simulink model "EKF"  (R2023b)
settings: Solver=FixedStepAuto  StartTime=tstart  StopTime=tend  FixedStep=0.1  RelTol=1e-3
values from neighbouring files (symbols this model uses):
  EKF_P0 = eye(7)    [main_script.m]
  inertia_p = [85.075, 0, 0; 0, 85.075, 0; 0, 0, 120.2515]    [omega_dot.m]
settings Model: Creator=Anna  LastModifiedBy=Ethan

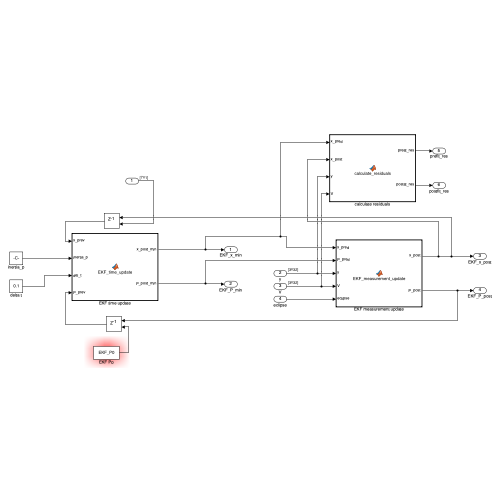
[thumbnail: Simulink's stored preview of the top-level diagram]
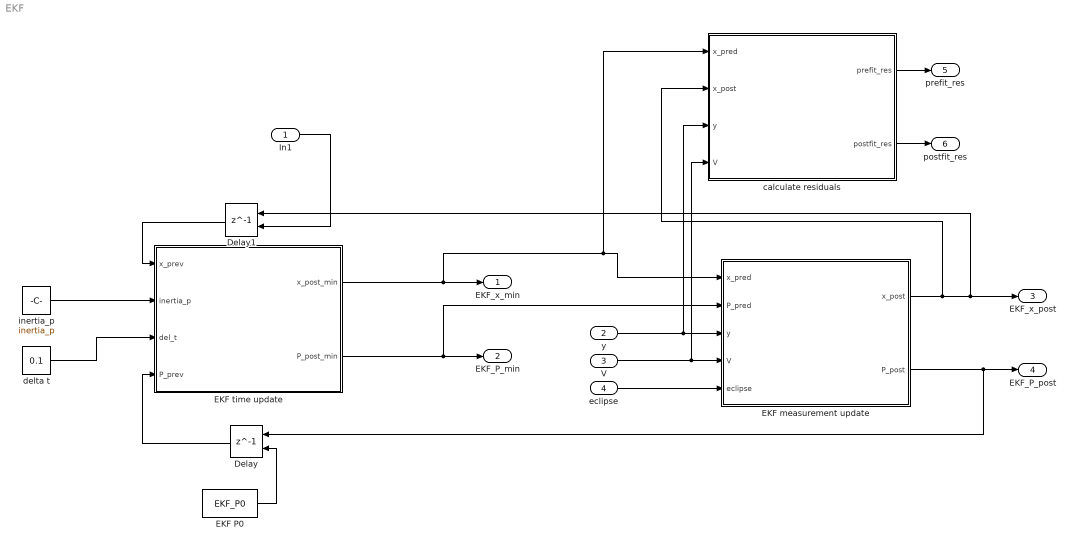
== system EKF ==
  In1 : Inport  PortDimensions=[7 1]
  y : Inport  Port=2  PortDimensions=[3, 32]
  V : Inport  Port=3  PortDimensions=[3, 32]
  eclipse : Inport  Port=4
  Delay : Delay  DelayLength=1  InitialConditionSource=Input port  InitialCondition=0
      settings: InputPortMap=u0,p4
  Delay1 : Delay  DelayLength=1  InitialConditionSource=Input port  InitialCondition=0
      settings: InputPortMap=u0,p4
  EKF P0 : Constant  Value=EKF_P0
  EKF measurement update : MATLAB Function  TreatAsAtomicUnit=on
  EKF time update : MATLAB Function  TreatAsAtomicUnit=on
  calculate residuals : MATLAB Function  TreatAsAtomicUnit=on
  delta t : Constant  Value=0.1
  inertia_p : Constant  Value=inertia_p
  EKF_x_min : Outport
  EKF_P_min : Outport  Port=2
  EKF_x_post : Outport  Port=3
  EKF_P_post : Outport  Port=4
  prefit_res : Outport  Port=5
  postfit_res : Outport  Port=6
  wires:
  Delay1/1 -> EKF time update/1(x_prev)
  In1/1 -> Delay1/2
  Delay/1 -> EKF time update/4(P_prev)
  EKF time update/1(x_post_min) -> calculate residuals/1(x_pred), EKF measurement update/1(x_pred), EKF_x_min/1
  EKF time update/2(P_post_min) -> EKF measurement update/2(P_pred), EKF_P_min/1
  EKF P0/1 -> Delay/2
  inertia_p/1 -> EKF time update/2(inertia_p)
  delta t/1 -> EKF time update/3(del_t)
  EKF measurement update/1(x_post) -> calculate residuals/2(x_post), Delay1/1, EKF_x_post/1
  EKF measurement update/2(P_post) -> Delay/1, EKF_P_post/1
  y/1 -> calculate residuals/3(y), EKF measurement update/3(y)
  V/1 -> calculate residuals/4(V), EKF measurement update/4(V)
  eclipse/1 -> EKF measurement update/5(eclipse)
  calculate residuals/1(prefit_res) -> prefit_res/1
  calculate residuals/2(postfit_res) -> postfit_res/1

== matlab function EKF/EKF measurement update ==
  data: x_pred input; P_pred input; y input; x_post output; P_post output; V input; eclipse input
function [x_post, P_post] = EKF_measurement_update(x_pred, P_pred, y, V, eclipse)

    

    %Sun
    if 1 %~eclipse
        rx = V(1, 1);
        ry = V(2, 1);
        rz = V(3, 1);
        q1 = x_pred(4);
        q2 = x_pred(5);
        q3 = x_pred(6);
        q4 = x_pred(7);
        
        %DCM 
        DCM = [q1^2 - q2^2 - q3^2 + q4^2, 2*q1*q2 + 2*q3*q4, 2*q1*q3 - 2*q2*q4;
            2*q1*q2 - 2*q3*q4, -q1^2 + q2^2 - q3^2 + q4^2, 2*q1*q4 + 2*q2*q3;
            2*q1*q3 + 2*q2*q4, 2*q2*q3 - 2*q1*q4, -q1^2 - q2^2 + q3^2 + q4^2];

        %Sensitivity Matrix
        H = [0, 0, 0, 2*q1*rx + 2*q2*ry + 2*q3*rz, -2*q2*rx + 2*q1*ry - 2*q4*rz, -2*q3*rx + 2*q4*ry + 2*q1*rz,  2*q4*rx + 2*q3*ry - 2*q2*rz;
            0, 0, 0, 2*q2*rx - 2*q1*ry + 2*q4*rz,  2*q1*rx + 2*q2*ry + 2*q3*rz, -2*q4*rx - 2*q3*ry + 2*q2*rz, -2*q3*rx + 2*q4*ry + 2*q1*rz;
            0, 0, 0, 2*q3*rx - 2*q4*ry - 2*q1*rz,  2*q4*rx + 2*q3*ry - 2*q2*rz,  2*q1*rx + 2*q2*ry + 2*q3*rz,  2*q2*rx - 2*q1*ry + 2*q4*rz];
        %Kalman Gain
        R = 0.13913 * eye(3);
        S = H * P_pred * H' + R;
        K = (P_pred * H')/(S); %nxm

        %disp(y(:, 1) - H * x_pred)
        x_pred = x_pred + K * (y(:, 1) -  DCM * V(:, 1));
        P_pred = (eye(length(x_pred), length(x_pred)) - K * H) * P_pred *(eye(length(x_pred), length(x_pred)))' + K*R*K';
 
    end
    
    %Magnetic
    rx = V(1, 2);
    ry = V(2, 2);
    rz = V(3, 2);
    q1 = x_pred(4);
    q2 = x_pred(5);
    q3 = x_pred(6);
    q4 = x_pred(7);

    %DCM 
    DCM = [q1^2 - q2^2 - q3^2 + q4^2, 2*q1*q2 + 2*q3*q4, 2*q1*q3 - 2*q2*q4;
            2*q1*q2 - 2*q3*q4, -q1^2 + q2^2 - q3^2 + q4^2, 2*q1*q4 + 2*q2*q3;
            2*q1*q3 + 2*q2*q4, 2*q2*q3 - 2*q1*q4, -q1^2 - q2^2 + q3^2 + q4^2];

    %Sensitivity Matrix
    H = [0, 0, 0, 2*q1*rx + 2*q2*ry + 2*q3*rz, -2*q2*rx + 2*q1*ry - 2*q4*rz, -2*q3*rx + 2*q4*ry + 2*q1*rz,  2*q4*rx + 2*q3*ry - 2*q2*rz;
        0, 0, 0, 2*q2*rx - 2*q1*ry + 2*q4*rz,  2*q1*rx + 2*q2*ry + 2*q3*rz, -2*q4*rx - 2*q3*ry + 2*q2*rz, -2*q3*rx + 2*q4*ry + 2*q1*rz;
        0, 0, 0, 2*q3*rx - 2*q4*ry - 2*q1*rz,  2*q4*rx + 2*q3*ry - 2*q2*rz,  2*q1*rx + 2*q2*ry + 2*q3*rz,  2*q2*rx - 2*q1*ry + 2*q4*rz];
    %Kalman Gain
    R =  3.05974 * 1e-7 * eye(3);
    S = H * P_pred * H' + R;
    K = (P_pred * H') / S; %nxm

    x_pred = x_pred + K * (y(:, 2) - DCM * V(:, 2));
    P_pred = (eye(length(x_pred), length(x_pred)) - K * H) * P_pred *(eye(length(x_pred), length(x_pred)))' + K*R*K';

    %Star
    for i = 3:32
        rx = V(1, i);
        ry = V(2, i);
        rz = V(3, i);
        q1 = x_pred(4);
        q2 = x_pred(5);
        q3 = x_pred(6);
        q4 = x_pred(7);


        %DCM 
        DCM = [q1^2 - q2^2 - q3^2 + q4^2, 2*q1*q2 + 2*q3*q4, 2*q1*q3 - 2*q2*q4;
                2*q1*q2 - 2*q3*q4, -q1^2 + q2^2 - q3^2 + q4^2, 2*q1*q4 + 2*q2*q3;
                2*q1*q3 + 2*q2*q4, 2*q2*q3 - 2*q1*q4, -q1^2 - q2^2 + q3^2 + q4^2];

        %Sensitivity Matrix
        H = [0, 0, 0, 2*q1*rx + 2*q2*ry + 2*q3*rz, -2*q2*rx + 2*q1*ry - 2*q4*rz, -2*q3*rx + 2*q4*ry + 2*q1*rz,  2*q4*rx + 2*q3*ry - 2*q2*rz;
            0, 0, 0, 2*q2*rx - 2*q1*ry + 2*q4*rz,  2*q1*rx + 2*q2*ry + 2*q3*rz, -2*q4*rx - 2*q3*ry + 2*q2*rz, -2*q3*rx + 2*q4*ry + 2*q1*rz;
            0, 0, 0, 2*q3*rx - 2*q4*ry - 2*q1*rz,  2*q4*rx + 2*q3*ry - 2*q2*rz,  2*q1*rx + 2*q2*ry + 2*q3*rz,  2*q2*rx - 2*q1*ry + 2*q4*rz];
        %Kalman Gain
        R = 2.342 * 1e-7 * eye(3);
        S = H * P_pred * H' + R;
        K = (P_pred * H') / S; %nxm



        x_pred = x_pred + K * (y(:, i) -  DCM * V(:, i));
        P_pred = (eye(length(x_pred), length(x_pred)) - K * H) * P_pred *(eye(length(x_pred), length(x_pred)))' + K*R*K';
    end
    
    x_post = x_pred;
    x_post(4:end) = x_post(4:end)./norm(x_post(4:end));
    P_post = P_pred;

== matlab function EKF/calculate residuals ==
  data: x_pred input; x_post input; prefit_res output; postfit_res output; y input; V input
function [prefit_res, postfit_res] = calculate_residuals(x_pred, x_post, y, V)
    prefit_res = zeros(3, 3);
    postfit_res = zeros(3, 3);
    
    %% Prefit
    q1 = x_pred(4);
    q2 = x_pred(5);
    q3 = x_pred(6);
    q4 = x_pred(7);

    rx = V(1, 1);
    ry = V(2, 1);
    rz = V(3, 1);

    %% Sun
    %DCM 
    DCM = [q1^2 - q2^2 - q3^2 + q4^2, 2*q1*q2 + 2*q3*q4, 2*q1*q3 - 2*q2*q4;
        2*q1*q2 - 2*q3*q4, -q1^2 + q2^2 - q3^2 + q4^2, 2*q1*q4 + 2*q2*q3;
        2*q1*q3 + 2*q2*q4, 2*q2*q3 - 2*q1*q4, -q1^2 - q2^2 + q3^2 + q4^2];

    %Sensitivity Matrix
    H = [0, 0, 0, 2*q1*rx + 2*q2*ry + 2*q3*rz, -2*q2*rx + 2*q1*ry - 2*q4*rz, -2*q3*rx + 2*q4*ry + 2*q1*rz,  2*q4*rx + 2*q3*ry - 2*q2*rz;
        0, 0, 0, 2*q2*rx - 2*q1*ry + 2*q4*rz,  2*q1*rx + 2*q2*ry + 2*q3*rz, -2*q4*rx - 2*q3*ry + 2*q2*rz, -2*q3*rx + 2*q4*ry + 2*q1*rz;
        0, 0, 0, 2*q3*rx - 2*q4*ry - 2*q1*rz,  2*q4*rx + 2*q3*ry - 2*q2*rz,  2*q1*rx + 2*q2*ry + 2*q3*rz,  2*q2*rx - 2*q1*ry + 2*q4*rz];
    %Kalman Gain
    prefit_res(:, 1) = y(:, 1) -  DCM * V(:, 1);

    
    %Magnetic
    rx = V(1, 2);
    ry = V(2, 2);
    rz = V(3, 2);

    %DCM 
    DCM = [q1^2 - q2^2 - q3^2 + q4^2, 2*q1*q2 + 2*q3*q4, 2*q1*q3 - 2*q2*q4;
            2*q1*q2 - 2*q3*q4, -q1^2 + q2^2 - q3^2 + q4^2, 2*q1*q4 + 2*q2*q3;
            2*q1*q3 + 2*q2*q4, 2*q2*q3 - 2*q1*q4, -q1^2 - q2^2 + q3^2 + q4^2];

    %Sensitivity Matrix
    H = [0, 0, 0, 2*q1*rx + 2*q2*ry + 2*q3*rz, -2*q2*rx + 2*q1*ry - 2*q4*rz, -2*q3*rx + 2*q4*ry + 2*q1*rz,  2*q4*rx + 2*q3*ry - 2*q2*rz;
        0, 0, 0, 2*q2*rx - 2*q1*ry + 2*q4*rz,  2*q1*rx + 2*q2*ry + 2*q3*rz, -2*q4*rx - 2*q3*ry + 2*q2*rz, -2*q3*rx + 2*q4*ry + 2*q1*rz;
        0, 0, 0, 2*q3*rx - 2*q4*ry - 2*q1*rz,  2*q4*rx + 2*q3*ry - 2*q2*rz,  2*q1*rx + 2*q2*ry + 2*q3*rz,  2*q2*rx - 2*q1*ry + 2*q4*rz];
    %Kalman Gain
    prefit_res(:, 2) = y(:, 2) -  DCM * V(:, 2);

    %Star
    star_residuals = zeros(3, 30);
    for i = 3:32
        rx = V(1, i);
        ry = V(2, i);
        rz = V(3, i);


        %DCM 
        DCM = [q1^2 - q2^2 - q3^2 + q4^2, 2*q1*q2 + 2*q3*q4, 2*q1*q3 - 2*q2*q4;
                2*q1*q2 - 2*q3*q4, -q1^2 + q2^2 - q3^2 + q4^2, 2*q1*q4 + 2*q2*q3;
                2*q1*q3 + 2*q2*q4, 2*q2*q3 - 2*q1*q4, -q1^2 - q2^2 + q3^2 + q4^2];

        %Sensitivity Matrix
        H = [0, 0, 0, 2*q1*rx + 2*q2*ry + 2*q3*rz, -2*q2*rx + 2*q1*ry - 2*q4*rz, -2*q3*rx + 2*q4*ry + 2*q1*rz,  2*q4*rx + 2*q3*ry - 2*q2*rz;
            0, 0, 0, 2*q2*rx - 2*q1*ry + 2*q4*rz,  2*q1*rx + 2*q2*ry + 2*q3*rz, -2*q4*rx - 2*q3*ry + 2*q2*rz, -2*q3*rx + 2*q4*ry + 2*q1*rz;
            0, 0, 0, 2*q3*rx - 2*q4*ry - 2*q1*rz,  2*q4*rx + 2*q3*ry - 2*q2*rz,  2*q1*rx + 2*q2*ry + 2*q3*rz,  2*q2*rx - 2*q1*ry + 2*q4*rz];
        %Kalman Gain
        star_residuals(:, i-2) = y(:, i) -  DCM * V(:, i);

    end
    prefit_res(:, 3) = mean(star_residuals, 2);

    %% Post fit

    q1 = x_post(4);
    q2 = x_post(5);
    q3 = x_post(6);
    q4 = x_post(7);
    %% Sun
    %DCM 
    DCM = [q1^2 - q2^2 - q3^2 + q4^2, 2*q1*q2 + 2*q3*q4, 2*q1*q3 - 2*q2*q4;
        2*q1*q2 - 2*q3*q4, -q1^2 + q2^2 - q3^2 + q4^2, 2*q1*q4 + 2*q2*q3;
        2*q1*q3 + 2*q2*q4, 2*q2*q3 - 2*q1*q4, -q1^2 - q2^2 + q3^2 + q4^2];

    %Sensitivity Matrix
    H = [0, 0, 0, 2*q1*rx + 2*q2*ry + 2*q3*rz, -2*q2*rx + 2*q1*ry - 2*q4*rz, -2*q3*rx + 2*q4*ry + 2*q1*rz,  2*q4*rx + 2*q3*ry - 2*q2*rz;
        0, 0, 0, 2*q2*rx - 2*q1*ry + 2*q4*rz,  2*q1*rx + 2*q2*ry + 2*q3*rz, -2*q4*rx - 2*q3*ry + 2*q2*rz, -2*q3*rx + 2*q4*ry + 2*q1*rz;
        0, 0, 0, 2*q3*rx - 2*q4*ry - 2*q1*rz,  2*q4*rx + 2*q3*ry - 2*q2*rz,  2*q1*rx + 2*q2*ry + 2*q3*rz,  2*q2*rx - 2*q1*ry + 2*q4*rz];
    %Kalman Gain
    postfit_res(:, 1) = y(:, 1) -  DCM * V(:, 1);

    
    %Magnetic
    rx = V(1, 2);
    ry = V(2, 2);
    rz = V(3, 2);

    %DCM 
    DCM = [q1^2 - q2^2 - q3^2 + q4^2, 2*q1*q2 + 2*q3*q4, 2*q1*q3 - 2*q2*q4;
            2*q1*q2 - 2*q3*q4, -q1^2 + q2^2 - q3^2 + q4^2, 2*q1*q4 + 2*q2*q3;
            2*q1*q3 + 2*q2*q4, 2*q2*q3 - 2*q1*q4, -q1^2 - q2^2 + q3^2 + q4^2];

    %Sensitivity Matrix
    H = [0, 0, 0, 2*q1*rx + 2*q2*ry + 2*q3*rz, -2*q2*rx + 2*q1*ry - 2*q4*rz, -2*q3*rx + 2*q4*ry + 2*q1*rz,  2*q4*rx + 2*q3*ry - 2*q2*rz;
        0, 0, 0, 2*q2*rx - 2*q1*ry + 2*q4*rz,  2*q1*rx + 2*q2*ry + 2*q3*rz, -2*q4*rx - 2*q3*ry + 2*q2*rz, -2*q3*rx + 2*q4*ry + 2*q1*rz;
        0, 0, 0, 2*q3*rx - 2*q4*ry - 2*q1*rz,  2*q4*rx + 2*q3*ry - 2*q2*rz,  2*q1*rx + 2*q2*ry + 2*q3*rz,  2*q2*rx - 2*q1*ry + 2*q4*rz];
    %Kalman Gain
    postfit_res(:, 2) = y(:, 2) -  DCM * V(:, 2);

    %Star
    star_residuals = zeros(3, 30);
    for i = 3:32
        rx = V(1, i);
        ry = V(2, i);
        rz = V(3, i);

        %DCM 
        DCM = [q1^2 - q2^2 - q3^2 + q4^2, 2*q1*q2 + 2*q3*q4, 2*q1*q3 - 2*q2*q4;
                2*q1*q2 - 2*q3*q4, -q1^2 + q2^2 - q3^2 + q4^2, 2*q1*q4 + 2*q2*q3;
                2*q1*q3 + 2*q2*q4, 2*q2*q3 - 2*q1*q4, -q1^2 - q2^2 + q3^2 + q4^2];

        %Sensitivity Matrix
        H = [0, 0, 0, 2*q1*rx + 2*q2*ry + 2*q3*rz, -2*q2*rx + 2*q1*ry - 2*q4*rz, -2*q3*rx + 2*q4*ry + 2*q1*rz,  2*q4*rx + 2*q3*ry - 2*q2*rz;
            0, 0, 0, 2*q2*rx - 2*q1*ry + 2*q4*rz,  2*q1*rx + 2*q2*ry + 2*q3*rz, -2*q4*rx - 2*q3*ry + 2*q2*rz, -2*q3*rx + 2*q4*ry + 2*q1*rz;
            0, 0, 0, 2*q3*rx - 2*q4*ry - 2*q1*rz,  2*q4*rx + 2*q3*ry - 2*q2*rz,  2*q1*rx + 2*q2*ry + 2*q3*rz,  2*q2*rx - 2*q1*ry + 2*q4*rz];
        %Kalman Gain
        star_residuals(:, i-2) = y(:, i) -  DCM * V(:, i);

    end
    postfit_res(:, 3) = mean(star_residuals, 2);

== matlab function EKF/EKF time update ==
  data: x_prev input; inertia_p input; del_t input; P_prev input; x_post_min output; P_post_min output
function [x_post_min, P_post_min] = EKF_time_update(x_prev,inertia_p, del_t, P_prev)
    %disp(x_prev)
    wx = x_prev(1);
    wy = x_prev(2);
    wz = x_prev(3);
    q1 = x_prev(4);
    q2 = x_prev(5);
    q3 = x_prev(6);
    q4 = x_prev(7);


    om = norm(x_prev(1:3));
    k = 1/om * sin(om * del_t/2);

    phi = zeros([7,7]); %state transition matrix
    phi(1:3, 1:3) = [1, (inertia_p(2,2) - inertia_p(3,3))/inertia_p(1,1) * x_prev(3)*del_t, (inertia_p(2,2) - inertia_p(3,3))/inertia_p(1,1) * x_prev(2)*del_t;
        (inertia_p(3,3) -inertia_p(1,1))/inertia_p(2,2) * x_prev(3) * del_t, 1, (inertia_p(3,3) -inertia_p(1,1))/inertia_p(2,2) * x_prev(1) * del_t;
        (inertia_p(1,1) -inertia_p(2,2))/inertia_p(3,3) * x_prev(2) * del_t, (inertia_p(1,1) -inertia_p(2,2))/inertia_p(3,3) * x_prev(1) * del_t, 1];
    phi(4:end, :) = [k*q4, -k*q3, k*q2, cos(om*del_t/2), k*wz, -k*wy, k*wx;
                    k*q3, k*q4, -k*q1, -k*wz, cos(om*del_t/2), k*wx, k*wy;
                    -k*q2, k*q1, k*q4, k*wy, -k*wx, cos(om*del_t/2), k*wz;
                    -k*q1, -k*q2, -k*q3, -k*wx, -k*wy, -k*wz, cos(om*del_t/2)];


    phi(4:7, 1:3) = [q4, -q3, q2;
                    q3, q4, -q1;
                   -q2, q1, q4;
                    -q1, -q2, -q3];
    Q = 1/1000 .* eye(7); %process noise
    x_post_min = phi * x_prev;
    P_post_min = phi * P_prev * phi' + Q;
